simulink model "Loop_detailed_model_v11_bipolar"  (R2013a)
settings: Solver=ode3  SolverMode=SingleTasking  StartTime=0.0  StopTime=4e-3  FixedStep=FS/50  MaxStep=1e-4  RelTol=1e-3
InitFcn:
  | %%%%%%  set scope time range
  | T_STOP=str2num(get_param(gcs,'StopTime'));
  | if numel(T_STOP) > 1
  |    T_STOP=T_STOP(2);
  | else
  |    T_STOP=T_STOP(1);
  | end
  | T_STOP=num2str(T_STOP);
  | 
  | %%%%%%  set scope time range in system @init_callback_fct
  | T_STOP=num2str(str2num(get_param(gcs,'StopTime')));
  | 
  | childs = allchild(0);
  | sol=strfind(upper(get(allchild(0),'Tag')),'VIEWER_PARAMETERS');
  | 
  | if iscell(sol)
  |    ind=find(~cellfun(@isempty, strfind(upper(get(allchild(0),'Tag')),'VIEWER_PARAMETERS')));
  | else
  |    ind=sol;
  | end
  | %ind=find(~cellfun(@isempty, {strfind(upper(get(allchild(0),'Tag')),'VIEWER_PARAMETERS'),[]}))
  | if ~isempty(ind)
  |    for k=1:length(childs(ind))
  |       set_param(getfield(get(childs(ind(k)),'UserData'),'block'),'TimeRange', T_STOP);
  | %      get_param(getfield(get(childs(ind(k)),'UserData'),'block'),'TimeRange');
  | %    set_param(getfield(get(childs(ind),'UserData'),'block'),'TimeRange',T_STOP);
  | %    get_param(getfield(get(childs(ind),'UserData'),'block'),'TimeRange');
  |    end
  | else
  |     warning(sprintf('VIEWER_PARAMETERS object not found\nOpen the config dialog by hand for the first sim start'))
  | end
undefined symbols (not defined in the file or in its folder): FS, Lc, Rc, Rsh, T1
libraries: simulink x3
settings Model: BufferReuse=off  Creator=mainster  LastModifiedBy=mainster
settings SolverCC: AutoInsertRateTranBlk=on
settings OptimizationCC: InlineParams=on  BufferReuse=off
settings DebuggingCC: InitInArrayFormatMsg=none
settings HardwareCC: ProdLargestAtomicInteger=Long  ProdLargestAtomicFloat=Double  ProdEndianess=LittleEndian  ProdHWDeviceType=ARM Compatible->ARM Cortex

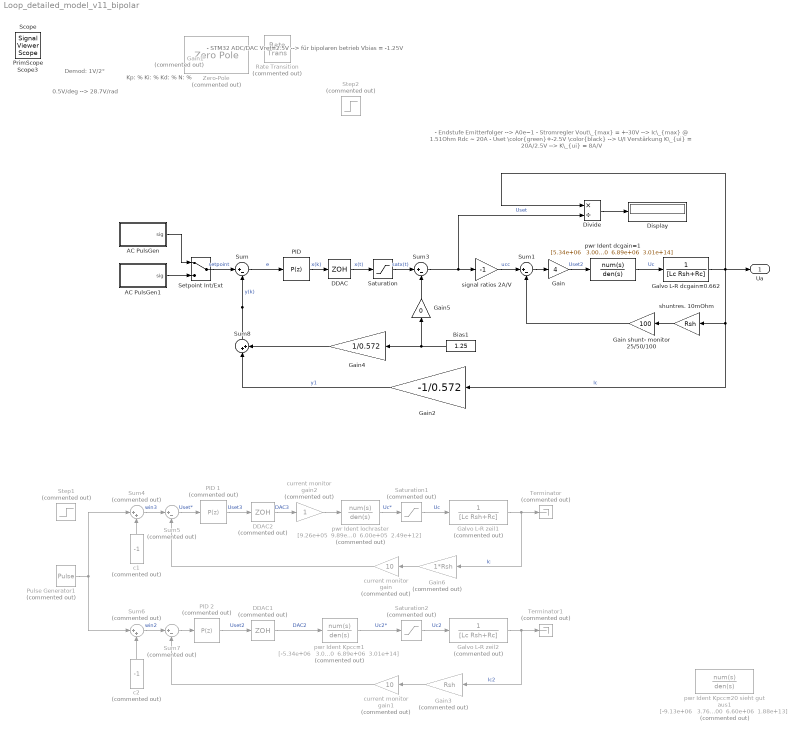
== system Loop_detailed_model_v11_bipolar ==
  note: - Endstufe Emitterfolger --> A0e~1
      | - Stromregler Vout\_{max} = +-30V
      |       --> Ic\_{max} @ 1.51Ohm Rdc ~ 20A
      | - Uset \color{green}+-2.5V \color{black}
      |       --> U/I Verstärkung K\_{ui} = 20A/2.5V
      |       --> K\_{ui} = 8A/V
  note: - STM32 ADC/DAC Vref=2.5V
      | --> für bipolaren betrieb Vbias = -1.25V
  note: Kp: % Ki: % Kd: % N: %
  note: 0.5V/deg --> 28.7V/rad
  note: Demod:
      | 1V/2°
  AC PulsGen : Subsystem  mask{sigp=0.5, sigpp=0, offs=1.25, peri=1e-3, duty=50}
      mask prompts: sigp "Insert signal peak"; sigpp "or signal peak-to-peak"; offs "Insert DC offset"; peri "periode"; duty "duty cycle in %"
      mask TypeOptions sigp: PulsGen/Amplitude
      mask Callback sigp:
      | %sigp=get_param([gcb '/PulsGen'],'Amplitude')
      | %SigVal=2*sigp
      mask TypeOptions offs: offset/Value
      mask TypeOptions peri: PulsGen/Period
      mask Display:
      | %str=sprintf('%s',get(gcbh,'ModelName'));
      | port_label('output', 1, '','texmode','off')
      | %text(.05,.98,['{\fontsize{12}\it\bf' strrep(str,'_',' ') '}'],'horizontalAlignment','left','verticalAlignment','top','texmode','on')
      | %text(.5,0.95,['{\fontsize{8}A_{peak}=}'],'horizontalAlignment','center','verticalAlignment','top','texmode','on')
      | disp(sprintf('Up=%.3g\nDC=%.3g',sigp, offs))
      | %disp(['Upp=' sigpp])%, offs))
      | %sprintf('sigpp==%s',sigpp)
      | %text(.15,.05,['{\fontsize{10}\itmechanics}'],'horizontalAlignment','left','verticalAlignment','bottom','texmode','on')
  AC PulsGen1 : Subsystem  mask{sigp=0.5, sigpp=0, offs=0}
      mask prompts: sigp "Insert signal peak"; sigpp "or signal peak-to-peak"; offs "Insert DC offset"
      mask TypeOptions sigp: PulsGen/Amplitude
      mask Callback sigp:
      | %sigp=get_param([gcb '/PulsGen'],'Amplitude')
      | %SigVal=2*sigp
      mask TypeOptions offs: offset/Value
      mask Display:
      | %str=sprintf('%s',get(gcbh,'ModelName'));
      | port_label('output', 1, '','texmode','off')
      | %text(.05,.98,['{\fontsize{12}\it\bf' strrep(str,'_',' ') '}'],'horizontalAlignment','left','verticalAlignment','top','texmode','on')
      | %text(.5,0.95,['{\fontsize{8}A_{peak}=}'],'horizontalAlignment','center','verticalAlignment','top','texmode','on')
      | disp(sprintf('Up=%.3g\nDC=%.3g',sigp, offs))
      | %disp(['Upp=' sigpp])%, offs))
      | %sprintf('sigpp==%s',sigpp)
      | %text(.15,.05,['{\fontsize{10}\itmechanics}'],'horizontalAlignment','left','verticalAlignment','bottom','texmode','on')
  Bias1 : Constant  Value=1.25  OutDataTypeStr=double  SampleTime=0
  DDAC : ZeroOrderHold  SampleTime=FS
      settings: AttributesFormatString=%<SampleTime>
  DDAC1 : ZeroOrderHold  Commented=on  SampleTime=FS
      settings: AttributesFormatString=%<SampleTime>
  DDAC2 : ZeroOrderHold  Commented=on  SampleTime=FS
      settings: AttributesFormatString=%<SampleTime>
  Display : Display
  Divide : Product  Inputs=*/
  Gain : Gain  Gain=4
  Gain shunt- monitor 25/50/100 : Gain  Gain=100
  Gain1 : Gain  Commented=on  Gain=2
  Gain2 : Gain  Gain=-1/0.572
  Gain3 : Gain  Commented=on  Gain=Rsh
  Gain4 : Gain  Gain=1/0.572
  Gain5 : Gain  Gain=0
  Gain6 : Gain  Commented=on  Gain=1*Rsh
  Galvo L-R dcgain=0.662 : TransferFcn  Numerator=1  Denominator=[Lc Rsh+Rc]
  Galvo L-R zeil1 : TransferFcn  Commented=on  Numerator=1  Denominator=[Lc Rsh+Rc]
  Galvo L-R zeil2 : TransferFcn  Commented=on  Numerator=1  Denominator=[Lc Rsh+Rc]
  "PID " : simulink/Continuous/PID Controller  Controller=P  TimeDomain=Discrete-time  SampleTime=FS  IntegratorMethod=Forward Euler  FilterMethod=Forward Euler  Form=Parallel  P=5  I=8149.05991185772  D=9.0248898483108e-05  N=10930.7783722874  InitialConditionSource=internal  InitialConditionForIntegrator=0  InitialConditionForFilter=0  ExternalReset=none  LimitOutput=off  UpperSaturationLimit=1.25  LowerSaturationLimit=-1.25  LinearizeAsGain=on  AntiWindupMode=clamping  Kb=1  TrackingMode=off  Kt=1  PParamMin=[]  PParamMax=[]  IParamMin=[]  IParamMax=[]  DParamMin=[]  DParamMax=[]  NParamMin=[]  NParamMax=[]  KbParamMin=[]  KbParamMax=[]  KtParamMin=[]  KtParamMax=[]  POutMin=[]  POutMax=[]  IOutMin=[]  IOutMax=[]  DOutMin=[]  DOutMax=[]  NOutMin=[]  NOutMax=[]  KbOutMin=[]  KbOutMax=[]  KtOutMin=[]  KtOutMax=[]  IntegratorOutMin=[]  IntegratorOutMax=[]  FilterOutMin=[]  FilterOutMax=[]  SumOutMin=[]  SumOutMax=[]  SumI1OutMin=[]  SumI1OutMax=[]  SumI2OutMin=[]  SumI2OutMax=[]  SumI3OutMin=[]  SumI3OutMax=[]  SumDOutMin=[]  SumDOutMax=[]  SaturationOutMin=[]  SaturationOutMax=[]  IntegratorContinuousStateAttributes=''  IntegratorStateMustResolveToSignalObject=off  IntegratorRTWStateStorageClass=Auto  FilterContinuousStateAttributes=''  FilterStateMustResolveToSignalObject=off  FilterRTWStateStorageClass=Auto
      settings: AttributesFormatString=UpLim=%<UpperSaturationLimit>\nLoLim=%<LowerSaturationLimit>\nKp=%<P>
  PID 1 : simulink/Continuous/PID Controller  Commented=on  Controller=P  TimeDomain=Discrete-time  SampleTime=FS  IntegratorMethod=Forward Euler  FilterMethod=Forward Euler  Form=Parallel  P=25.2263389172728  I=3745.38790742202  D=9.0248898483108e-05  N=10930.7783722874  InitialConditionSource=internal  InitialConditionForIntegrator=0  InitialConditionForFilter=0  ExternalReset=none  LimitOutput=off  UpperSaturationLimit=1.25  LowerSaturationLimit=-1.25  LinearizeAsGain=on  AntiWindupMode=clamping  Kb=1  TrackingMode=off  Kt=1  PParamMin=[]  PParamMax=[]  IParamMin=[]  IParamMax=[]  DParamMin=[]  DParamMax=[]  NParamMin=[]  NParamMax=[]  KbParamMin=[]  KbParamMax=[]  KtParamMin=[]  KtParamMax=[]  POutMin=[]  POutMax=[]  IOutMin=[]  IOutMax=[]  DOutMin=[]  DOutMax=[]  NOutMin=[]  NOutMax=[]  KbOutMin=[]  KbOutMax=[]  KtOutMin=[]  KtOutMax=[]  IntegratorOutMin=[]  IntegratorOutMax=[]  FilterOutMin=[]  FilterOutMax=[]  SumOutMin=[]  SumOutMax=[]  SumI1OutMin=[]  SumI1OutMax=[]  SumI2OutMin=[]  SumI2OutMax=[]  SumI3OutMin=[]  SumI3OutMax=[]  SumDOutMin=[]  SumDOutMax=[]  SaturationOutMin=[]  SaturationOutMax=[]  IntegratorContinuousStateAttributes=''  IntegratorStateMustResolveToSignalObject=off  IntegratorRTWStateStorageClass=Auto  FilterContinuousStateAttributes=''  FilterStateMustResolveToSignalObject=off  FilterRTWStateStorageClass=Auto
  PID 2 : simulink/Continuous/PID Controller  Commented=on  Controller=P  TimeDomain=Discrete-time  SampleTime=FS  IntegratorMethod=Forward Euler  FilterMethod=Forward Euler  Form=Parallel  P=9.78763876336799  I=3745.38790742202  D=9.0248898483108e-05  N=10930.7783722874  InitialConditionSource=internal  InitialConditionForIntegrator=0  InitialConditionForFilter=0  ExternalReset=none  LimitOutput=off  UpperSaturationLimit=1.25  LowerSaturationLimit=-1.25  LinearizeAsGain=on  AntiWindupMode=clamping  Kb=1  TrackingMode=off  Kt=1  PParamMin=[]  PParamMax=[]  IParamMin=[]  IParamMax=[]  DParamMin=[]  DParamMax=[]  NParamMin=[]  NParamMax=[]  KbParamMin=[]  KbParamMax=[]  KtParamMin=[]  KtParamMax=[]  POutMin=[]  POutMax=[]  IOutMin=[]  IOutMax=[]  DOutMin=[]  DOutMax=[]  NOutMin=[]  NOutMax=[]  KbOutMin=[]  KbOutMax=[]  KtOutMin=[]  KtOutMax=[]  IntegratorOutMin=[]  IntegratorOutMax=[]  FilterOutMin=[]  FilterOutMax=[]  SumOutMin=[]  SumOutMax=[]  SumI1OutMin=[]  SumI1OutMax=[]  SumI2OutMin=[]  SumI2OutMax=[]  SumI3OutMin=[]  SumI3OutMax=[]  SumDOutMin=[]  SumDOutMax=[]  SaturationOutMin=[]  SaturationOutMax=[]  IntegratorContinuousStateAttributes=''  IntegratorStateMustResolveToSignalObject=off  IntegratorRTWStateStorageClass=Auto  FilterContinuousStateAttributes=''  FilterStateMustResolveToSignalObject=off  FilterRTWStateStorageClass=Auto
  Pulse Generator1 : DiscretePulseGenerator  Commented=on  PulseType=Time based  Amplitude=2  Period=4e-3  PulseWidth=50  SampleTime=FS
  Rate Transition : RateTransition  Commented=on  OutPortSampleTime=FS
  Saturation : Saturate  UpperLimit=125  LowerLimit=-125
      settings: AttributesFormatString=Up_lim=%<UpperLimit>\nLo_lim=%<LowerLimit>
  Saturation1 : Saturate  Commented=on  UpperLimit=30  LowerLimit=-30
      settings: AttributesFormatString=Up_lim=%<UpperLimit>\nLo_lim=%<LowerLimit>
  Saturation2 : Saturate  Commented=on  UpperLimit=30  LowerLimit=-30
      settings: AttributesFormatString=Up_lim=%<UpperLimit>\nLo_lim=%<LowerLimit>
  Setpoint Int/Ext : ManualSwitch  SampleTime=FS
  Step1 : Step  Commented=on  Time=2e-3  After=1.25  SampleTime=0
      settings: AttributesFormatString=Time:%<Time>\nAmp:%<After>
  Step2 : Step  Commented=on  Time=0  After=1.25  SampleTime=0
      settings: AttributesFormatString=Time:%<Time>\nAmp:%<After>
  Sum : Sum  Inputs=|+-  SampleTime=FS
  Sum1 : Sum  Inputs=|+-
  Sum3 : Sum  Inputs=|+-
  Sum4 : Sum  Commented=on  Inputs=|++  SampleTime=FS
  Sum5 : Sum  Commented=on  Inputs=|+-  SampleTime=FS
  Sum6 : Sum  Commented=on  Inputs=|++  SampleTime=FS
  Sum7 : Sum  Commented=on  Inputs=|+-  SampleTime=FS
  Sum8 : Sum  Inputs=|++
  Terminator : Terminator  Commented=on
  Terminator1 : Terminator  Commented=on
  Zero-Pole : ZeroPole  Commented=on  Zeros=[]  Poles=[-1/T1 -1/T1]  Gain=(1/T1)^2
  c1 : Constant  Commented=on  Value=-1  SampleTime=FS
  c2 : Constant  Commented=on  Value=-1  SampleTime=FS
  current monitor gain : Gain  Commented=on  Gain=10
  current monitor gain1 : Gain  Commented=on  Gain=10
  current monitor gain2 : Gain  Commented=on
  "pwr Ident Kpcc=1 " : TransferFcn  Commented=on  Numerator="[-5.34e+06   3.00e+14]"  Denominator="[1.00e+00  6.89e+06  3.01e+14]"
  pwr Ident dcgain=1 : TransferFcn  Numerator="[5.34e+06   3.00e+14]"  Denominator="[1.00e+00  6.89e+06  3.01e+14]"
  pwr Ident lochraster : TransferFcn  Commented=on  Numerator="[9.26e+05  9.89e+11]"  Denominator="[1.00e+00  6.00e+05  2.49e+12]"
  pwr Ident Kpcc=20 sieht gut aus1 : TransferFcn  Commented=on  Numerator="[-9.13e+06   3.76e+14]"  Denominator="[1.00e+00  6.60e+06  1.88e+13]"
  shuntres. 10mOhm : Gain  Gain=Rsh
  signal ratios 2A/V : Gain  Gain=-1
  Ua : Outport  SampleTime=FS
  PrimScope : SignalViewerScope  IOType=viewer  NumInputPorts=6  ZoomMode=yonly  LegendLocations=|  RefreshTime=0.035000
      | 0.81244     0.90024     0.16886    0.036879
      | 0.71487     0.76462     0.15898    0.036879
      | 0.77438     0.62345     0.13921    0.036879
      | 0.70296     0.44889     0.10956    0.020704
      | 0.78628     0.30771     0.16886    0.053054
      | 0.79818     0.14933     0.10956    0.020704
      settings: ShowLegends=on  TimeRange=0.008  YMin=0~-10~-40~0~-2~-40  YMax=2~5~40~1~3~40
  Scope : SignalViewerScope  IOType=viewer  RefreshTime=0.035000
  Scope3 : SignalViewerScope  IOType=viewer  ZoomMode=yonly  RefreshTime=0.035000
      settings: YMin=1  YMax=3  SaveName=ScopeData3
  wires:
  Sum/1 -> "PID "/1  "e"
  Galvo L-R dcgain=0.662/1 -> Divide/1, shuntres. 10mOhm/1, Gain2/1, Ua/1  "Ic"
  "PID "/1 -> DDAC/1  "x(k)"
  Sum8/1 -> Sum/2  "y(k)"
  Gain/1 -> pwr Ident dcgain=1/1  "Uset2"
  pwr Ident dcgain=1/1 -> Galvo L-R dcgain=0.662/1  "Uc"
  Saturation/1 -> Sum3/1  "satx(t)"
  Sum3/1 -> signal ratios 2A/V/1, Divide/2  "Uset"
  DDAC/1 -> Saturation/1  "x(t)"
  PID 1/1 -> DDAC2/1  "Uset3"
  pwr Ident lochraster/1 -> Saturation1/1  "Uc*"
  Galvo L-R zeil1/1 -> Gain6/1, Terminator/1  "Ic"
  Pulse Generator1/1 -> Sum6/1, Sum4/1
  c1/1 -> Sum4/2
  Sum4/1 -> Sum5/1  "win3"
  Sum5/1 -> PID 1/1  "Uset*"
  Saturation1/1 -> Galvo L-R zeil1/1  "Uc"
  Gain6/1 -> current monitor gain/1
  current monitor gain/1 -> Sum5/2
  PID 2/1 -> DDAC1/1  "Uset2"
  "pwr Ident Kpcc=1 "/1 -> Saturation2/1  "Uc2*"
  Galvo L-R zeil2/1 -> Gain3/1, Terminator1/1  "Ic2"
  c2/1 -> Sum6/2
  Sum6/1 -> Sum7/1  "win2"
  Sum7/1 -> PID 2/1
  Saturation2/1 -> Galvo L-R zeil2/1  "Uc2"
  Gain3/1 -> current monitor gain1/1
  current monitor gain1/1 -> Sum7/2
  DDAC1/1 -> "pwr Ident Kpcc=1 "/1  "DAC2"
  DDAC2/1 -> current monitor gain2/1  "DAC3"
  current monitor gain2/1 -> pwr Ident lochraster/1
  Setpoint Int/Ext/1 -> Sum/1  "setpoint"
  AC PulsGen/1(sig) -> Setpoint Int/Ext/1
  AC PulsGen1/1(sig) -> Setpoint Int/Ext/2
  Gain2/1 -> Sum8/1  "y1"
  Sum1/1 -> Gain/1
  Gain shunt- monitor 25/50/100/1 -> Sum1/2
  shuntres. 10mOhm/1 -> Gain shunt- monitor 25/50/100/1
  Divide/1 -> Display/1
  signal ratios 2A/V/1 -> Sum1/1  "ucc"
  Gain4/1 -> Sum8/2
  Bias1/1 -> Gain5/1, Gain4/1
  Gain5/1 -> Sum3/2

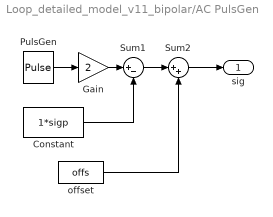
== system Loop_detailed_model_v11_bipolar/AC PulsGen ==
  Constant : Constant  Value=1*sigp
  Gain : Gain  Gain=2  SampleTime=FS
  PulsGen : DiscretePulseGenerator  PulseType=Time based  Amplitude=sigp  Period=peri  PulseWidth=50  PhaseDelay=0.5e-3  SampleTime=FS
      settings: AttributesFormatString=A=%<Amplitude>\nPeri=%<Period>
  Sum1 : Sum  Inputs=|+-  SampleTime=FS
  Sum2 : Sum  Inputs=|++  SampleTime=FS
  offset : Constant  Value=offs  SampleTime=FS
  sig : Outport
  wires:
  Sum2/1 -> sig/1
  PulsGen/1 -> Gain/1
  offset/1 -> Sum2/2
  Gain/1 -> Sum1/1
  Sum1/1 -> Sum2/1
  Constant/1 -> Sum1/2

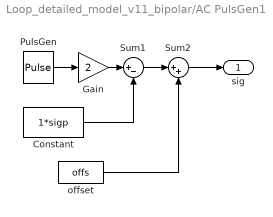
== system Loop_detailed_model_v11_bipolar/AC PulsGen1 ==
  Constant : Constant  Value=1*sigp
  Gain : Gain  Gain=2
  PulsGen : DiscretePulseGenerator  PulseType=Time based  Amplitude=sigp  Period=4e-3  PulseWidth=50  PhaseDelay=0.5e-3  SampleTime=FS
      settings: AttributesFormatString=A=%<Amplitude>\nPeri=%<Period>
  Sum1 : Sum  Inputs=|+-
  Sum2 : Sum  Inputs=|++
  offset : Constant  Value=offs
  sig : Outport
  wires:
  Sum2/1 -> sig/1
  PulsGen/1 -> Gain/1
  offset/1 -> Sum2/2
  Gain/1 -> Sum1/1
  Sum1/1 -> Sum2/1
  Constant/1 -> Sum1/2
